simulink model "Signal_Generator"  (Simulink 8.0)
settings: Solver=ode45  StartTime=0.0  StopTime=10.0  RelTol=1e-3
settings Model: Creator=Faradars  LastModifiedBy=Faradars

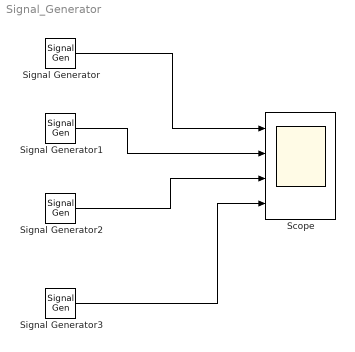
== system Signal_Generator ==
  Scope : Scope  NumInputPorts=4
      settings: TimeRange=10  YMin=-5~-5~-5~-5  YMax=5~5~5~5
  Signal Generator : SignalGenerator  Frequency=0.2
  Signal Generator1 : SignalGenerator  WaveForm=square  Frequency=0.2
  Signal Generator2 : SignalGenerator  WaveForm=sawtooth  Frequency=0.2
  Signal Generator3 : SignalGenerator  WaveForm=random  Frequency=0.2
  wires:
  Signal Generator/1 -> Scope/1
  Signal Generator1/1 -> Scope/2
  Signal Generator2/1 -> Scope/3
  Signal Generator3/1 -> Scope/4
